simulink model "DQReferenceCurrentCalculationComponent"  (R2025b)
settings: Solver=FixedStepDiscrete  StartTime=0.0  StopTime=10.0  RelTol=1e-3
undefined symbols (not defined in the file): D1, P
settings Model: OrderFunctionsByDependency=on  Creator=dakaihu  LastModifiedBy=dakaihu
settings OptimizationCC: DefaultParameterBehavior=Inlined  UseFloatMulNetSlope=on  EnhancedBackFolding=on  PassReuseOutputArgsAs=Individual arguments  ZeroExternalMemoryAtStartup=off  ZeroInternalMemoryAtStartup=off  OptimizeBlockOrder=speed  DifferentSizesBufferReuse=on  OptimizationCustomize=off  EfficientTunableParamExpr=on
settings DebuggingCC: ParameterTunabilityLossMsg=error
settings HardwareCC: ProdBitPerChar=16.0  ProdBitPerInt=16.0  ProdBitPerPointer=32.0  ProdBitPerSizeT=32.0  ProdBitPerPtrDiffT=32.0  ProdLargestAtomicInteger=Integer  ProdLargestAtomicFloat=None  ProdWordSize=16.0  ProdLongLongMode=on  ProdHWDeviceType=Texas Instruments->C2000
settings SFSimCC: MATLABDynamicMemAlloc=off
settings RTWCC: SystemTargetFile=ert.tlc  GenCodeOnly=on  TemplateMakefile=ert_default_tmf  Description=Embedded Coder
settings CodeAppCC: ForceParamTrailComments=on  IgnoreCustomStorageClasses=off  MaxIdLength=60.0  OperatorAnnotations=on  SimulinkDataObjDesc=on  SFDataObjDesc=on  InsertBlockDesc=on
settings ERTTargetCC: ERTCustomFileTemplate=example_file_process.tlc  TargetLangStandard=C99 (ISO)  GenerateSampleERTMain=on

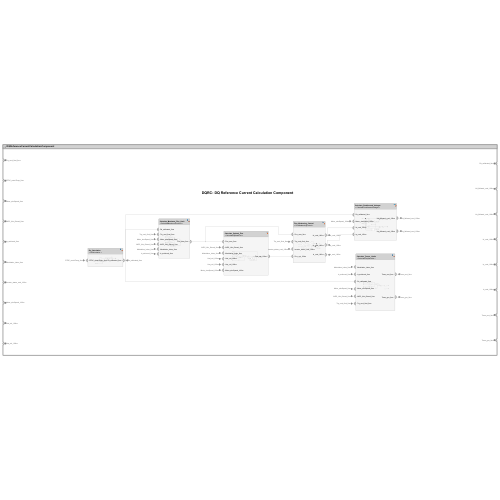
[thumbnail: Simulink's stored preview of the top-level diagram]
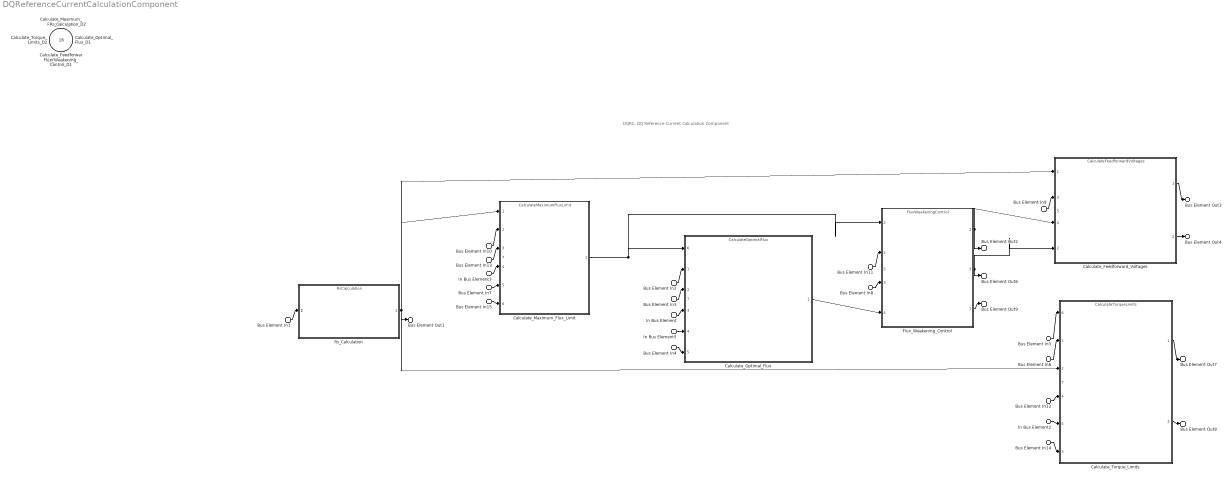
== system DQReferenceCurrentCalculationComponent ==
  note: DQRC: DQ Reference Current Calculation Component
  Bus Element In11 : Inport  RequirementInfo={} %GIDa_42953e8e_de57_4322_b6d3_fbe42e62adbf  PortName=Trq_cmd_final_2ms
  Bus Element In10 : Inport  RequirementInfo={} %GIDa_8c77aa49_9124_491b_8864_da37a441f5cb  PortName=Trq_cmd_final_2ms
  Bus Element In14 : Inport  RequirementInfo={} %GIDa_ea2f610a_4c5f_4cd4_9701_be585be16287  PortName=Trq_cmd_final_2ms
  Bus Element In1 : Inport  RequirementInfo={} %GIDa_4f0251a4_2495_47e1_b29c_9e0429a6851b  Port=2  PortName=STDC_motorTemp_2ms
  Bus Element In13 : Inport  RequirementInfo={} %GIDa_c753a603_7d00_42cf_be23_a4aecb64df4c  Port=3  PortName=Motor_elecSpeed_2ms
  Bus Element In12 : Inport  RequirementInfo={} %GIDa_cf1e9558_22e9_402c_a4b9_90f14ffe8b89  Port=3  PortName=Motor_elecSpeed_2ms
  In Bus Element3 : Inport  RequirementInfo={} %GIDa_41c1c28b_496d_4099_b24e_4d87927b0cd5  Port=4  PortName=IHDC_Vdc_filtered_2ms
  Bus Element In2 : Inport  RequirementInfo={} %GIDa_620fb42b_f1fb_400e_beea_66cdd1a5168a  Port=4  PortName=IHDC_Vdc_filtered_2ms
  In Bus Element2 : Inport  RequirementInfo={} %GIDa_a1449eb5_d98c_47be_a41f_d54f6146e101  Port=4  PortName=IHDC_Vdc_filtered_2ms
  Bus Element In6 : Inport  RequirementInfo={} %GIDa_46e95821_090d_4c5e_b6ae_42df5a77a427  Port=5  PortName=Is_achieved_2ms
  Bus Element In15 : Inport  RequirementInfo={} %GIDa_5aa52e8c_01f1_4417_9777_fe34b7f6ede0  Port=5  PortName=Is_achieved_2ms
  Bus Element In7 : Inport  RequirementInfo={} %GIDa_024a4306_83b0_46fe_af59_1f46b343fa8c  Port=6  PortName=Modulation_index_2ms
  Bus Element In3 : Inport  RequirementInfo={} %GIDa_be1195a5_2365_4ab0_90e8_c535b97f38fb  Port=6  PortName=Modulation_index_2ms
  Bus Element In5 : Inport  RequirementInfo={} %GIDa_dc760428_b6dc_4320_9a29_40c08d693f8a  Port=6  PortName=Modulation_index_2ms
  Bus Element In8 : Inport  RequirementInfo={} %GIDa_b12bee26_3679_4b52_8fa4_20643664e455  Port=7  PortName=Inverter_status_cmd_100us
  Bus Element In9 : Inport  RequirementInfo={} %GIDa_3f02f1c3_17f3_49f8_a464_eadd2057f829  Port=8  PortName=Motor_elecSpeed_100us
  Bus Element In4 : Inport  RequirementInfo={} %GIDa_8f5b8e9c_1d9d_4003_b734_3b70d64320b5  Port=8  PortName=Motor_elecSpeed_100us
  In Bus Element : Inport  RequirementInfo={} %GIDa_7ff0a437_48bf_41fa_8fef_4c1583c1267a  Port=9  PortName=Usd_ctrl_100us
  In Bus Element5 : Inport  RequirementInfo={} %GIDa_fb215a39_59d4_42c0_a18e_4b3e3a2c8f98  Port=10  PortName=Usq_ctrl_100us
  Calculate_Feedforward_Voltages_D1 : Inport  Port=11  OutputFunctionCall=on
  Calculate_Maximum_Flux_Limit_D2 : Inport  Port=12  OutputFunctionCall=on
  Calculate_Optimal_Flux_D1 : Inport  Port=13  OutputFunctionCall=on
  Calculate_Torque_Limits_D2 : Inport  Port=14  OutputFunctionCall=on
  Flux_Weakening_Control_D1 : Inport  Port=15  OutputFunctionCall=on
  Rs_Calculation_D2 : Inport  Port=16  OutputFunctionCall=on
  "Calculate_Feedforward_Voltages " : ModelReference  RequirementInfo={} %GIDa_c2d31358_4466_4952_b1b2_7ab47b6be7d3  ModelNameDialog=CalculateFeedforwardVoltages  SimulationMode=Normal  ScheduleRates=on  CachedPortDiscreteRates=[0.0001]  ModelEventPortInfo=P:D1[0.0001][0][0]  ModelReferenceVersion=2.2
      settings: PortSchema="{\"entries\":[{\"content\":{\"headerSize\":38,\"margin\":15,\"minimumSpacing\":25,\"sides\":[{\"content\":{\"connectorIds\":[\"In1\",\"In3\",\"In4\",\"In2\"]},\"type\":\"ConnectorPlacement.EquallySpacedRectSide\",\"uuid\":\"b2f30fca-3d8e-46ee-af1d-282b22b9b844\"},{\"content\":{\"connectorIds\":[\"Out1\",\"Out2\"],\"side\":\"RIGHT\"},\"type\":\"ConnectorPlacement.EquallySpacedRectSide\",\"uuid\":\"2d7d706d-eac4-4c73-84e8-2a36a393a616\"},{\"content\":{\"side\":\"TOP\"},\"type\":\"ConnectorPlacement.EquallySpacedRectSide\",\"uuid\":\"b52ae510-b7cc-4ed0-8d34-4a095deae41b\"},{\"content\":{\"side\":\"BOTTOM\"},\"type\":\"ConnectorPlacement.EquallySpacedRectSide\",\"uuid\":\"4f396a3e-469c-4bfe-8758-61b37cfc3b8b\"},{\"content\":{\"connectorIds\":[\"In5\"],\"side\":\"HIDDEN\"},\"type\":\"ConnectorPlacement.EquallySpacedRectSide\",\"uuid\":\"844b9219-0887-483b-96de-eb0af172b250\"}]},\"type\":\"ConnectorPlacement.EquallySpacedConnector\",\"uuid\":\"1257e7cc-1858-4bc4-ab05-7b00060cf0d5\"}],\"packageUris\":[\"http://schema.mathworks.com/mf0/Connector/R2020b\"],\"version\":\"1.0\"}"
  Calculate_Maximum_Flux_Limit : ModelReference  RequirementInfo={} %GIDa_a87a5d76_4785_45de_8980_7f650c5fa9a2  ModelNameDialog=CalculateMaximumFluxLimit  SimulationMode=Normal  ScheduleRates=on  CachedPortDiscreteRates=[0.002]  ModelEventPortInfo=P:D1[0.002][0][0]  ModelReferenceVersion=2.2
      settings: PortSchema="{\"entries\":[{\"content\":{\"headerSize\":38,\"margin\":15,\"minimumSpacing\":25,\"sides\":[{\"content\":{\"connectorIds\":[\"In1\",\"In2\",\"In3\",\"In4\",\"In5\",\"In6\"]},\"type\":\"ConnectorPlacement.EquallySpacedRectSide\",\"uuid\":\"b2f30fca-3d8e-46ee-af1d-282b22b9b844\"},{\"content\":{\"connectorIds\":[\"Out1\"],\"side\":\"RIGHT\"},\"type\":\"ConnectorPlacement.EquallySpacedRectSide\",\"uuid\":\"2d7d706d-eac4-4c73-84e8-2a36a393a616\"},{\"content\":{\"side\":\"TOP\"},\"type\":\"ConnectorPlacement.EquallySpacedRectSide\",\"uuid\":\"b52ae510-b7cc-4ed0-8d34-4a095deae41b\"},{\"content\":{\"connectorIds\":[\"In7\"],\"side\":\"HIDDEN\"},\"type\":\"ConnectorPlacement.EquallySpacedRectSide\",\"uuid\":\"d71c0094-66e8-4c46-a453-bb528cb08d1e\"}]},\"type\":\"ConnectorPlacement.EquallySpacedConnector\",\"uuid\":\"1257e7cc-1858-4bc4-ab05-7b00060cf0d5\"}],\"packageUris\":[\"http://schema.mathworks.com/mf0/Connector/R2020b\"],\"version\":\"1.0\"}"
  Calculate_Optimal_Flux : ModelReference  RequirementInfo={} %GIDa_8fb845d2_dc36_4fd4_9091_e75f493b384f  ModelNameDialog=CalculateOptimalFlux  SimulationMode=Normal  ScheduleRates=on  CachedPortDiscreteRates=[0.0001]  ModelEventPortInfo=P:D1[0.0001][0][0]  ModelReferenceVersion=2.2
      settings: PortSchema="{\"entries\":[{\"content\":{\"headerSize\":38,\"margin\":15,\"minimumSpacing\":25,\"sides\":[{\"content\":{\"connectorIds\":[\"In6\",\"In1\",\"In2\",\"In3\",\"In4\",\"In5\"]},\"type\":\"ConnectorPlacement.EquallySpacedRectSide\",\"uuid\":\"b2f30fca-3d8e-46ee-af1d-282b22b9b844\"},{\"content\":{\"connectorIds\":[\"Out1\"],\"side\":\"RIGHT\"},\"type\":\"ConnectorPlacement.EquallySpacedRectSide\",\"uuid\":\"2d7d706d-eac4-4c73-84e8-2a36a393a616\"},{\"content\":{\"side\":\"TOP\"},\"type\":\"ConnectorPlacement.EquallySpacedRectSide\",\"uuid\":\"b52ae510-b7cc-4ed0-8d34-4a095deae41b\"},{\"content\":{\"connectorIds\":[\"In7\"],\"side\":\"HIDDEN\"},\"type\":\"ConnectorPlacement.EquallySpacedRectSide\",\"uuid\":\"a73ad583-9615-4874-ab2d-c98618391765\"}]},\"type\":\"ConnectorPlacement.EquallySpacedConnector\",\"uuid\":\"1257e7cc-1858-4bc4-ab05-7b00060cf0d5\"}],\"packageUris\":[\"http://schema.mathworks.com/mf0/Connector/R2020b\"],\"version\":\"1.0\"}"
  Calculate_Torque_Limits : ModelReference  RequirementInfo={} %GIDa_739b0719_e4db_4236_85d1_8411d06b7a29  ModelNameDialog=CalculateTorqueLimits  SimulationMode=Normal  ScheduleRates=on  CachedPortDiscreteRates=[0.002]  ModelEventPortInfo=P:D1[0.002][0][0]  ModelReferenceVersion=2.2
      settings: PortSchema="{\"entries\":[{\"content\":{\"headerSize\":38,\"margin\":15,\"minimumSpacing\":25,\"sides\":[{\"content\":{\"connectorIds\":[\"In6\",\"In1\",\"In2\",\"In4\",\"In5\",\"In3\"]},\"type\":\"ConnectorPlacement.EquallySpacedRectSide\",\"uuid\":\"b2f30fca-3d8e-46ee-af1d-282b22b9b844\"},{\"content\":{\"connectorIds\":[\"Out1\",\"Out2\"],\"side\":\"RIGHT\"},\"type\":\"ConnectorPlacement.EquallySpacedRectSide\",\"uuid\":\"2d7d706d-eac4-4c73-84e8-2a36a393a616\"},{\"content\":{\"side\":\"TOP\"},\"type\":\"ConnectorPlacement.EquallySpacedRectSide\",\"uuid\":\"b52ae510-b7cc-4ed0-8d34-4a095deae41b\"},{\"content\":{\"connectorIds\":[\"In7\"],\"side\":\"HIDDEN\"},\"type\":\"ConnectorPlacement.EquallySpacedRectSide\",\"uuid\":\"bfe6c03f-982a-4b44-9f69-90b5c2e623cb\"}]},\"type\":\"ConnectorPlacement.EquallySpacedConnector\",\"uuid\":\"1257e7cc-1858-4bc4-ab05-7b00060cf0d5\"}],\"packageUris\":[\"http://schema.mathworks.com/mf0/Connector/R2020b\"],\"version\":\"1.0\"}"
  Flux_Weakening_Control : ModelReference  RequirementInfo={} %GIDa_9fe039aa_e028_435b_8ff1_3eb9542dc048  ModelNameDialog=FluxWeakeningControl  SimulationMode=Normal  ScheduleRates=on  CachedPortDiscreteRates=[0.0001]  ModelEventPortInfo=P:D1[0.0001][0][0]  ModelReferenceVersion=2.0
      settings: PortSchema="{\"entries\":[{\"content\":{\"headerSize\":38,\"margin\":15,\"minimumSpacing\":25,\"sides\":[{\"content\":{\"connectorIds\":[\"In2\",\"In1\",\"In3\",\"In4\"]},\"type\":\"ConnectorPlacement.EquallySpacedRectSide\",\"uuid\":\"b2f30fca-3d8e-46ee-af1d-282b22b9b844\"},{\"content\":{\"connectorIds\":[\"Out2\",\"Out3\",\"Out1\"],\"side\":\"RIGHT\"},\"type\":\"ConnectorPlacement.EquallySpacedRectSide\",\"uuid\":\"2d7d706d-eac4-4c73-84e8-2a36a393a616\"},{\"content\":{\"side\":\"TOP\"},\"type\":\"ConnectorPlacement.EquallySpacedRectSide\",\"uuid\":\"b52ae510-b7cc-4ed0-8d34-4a095deae41b\"},{\"content\":{\"connectorIds\":[\"In5\"],\"side\":\"HIDDEN\"},\"type\":\"ConnectorPlacement.EquallySpacedRectSide\",\"uuid\":\"7d4a66f0-dbef-49ea-acd8-9a102931ed07\"}]},\"type\":\"ConnectorPlacement.EquallySpacedConnector\",\"uuid\":\"1257e7cc-1858-4bc4-ab05-7b00060cf0d5\"}],\"packageUris\":[\"http://schema.mathworks.com/mf0/Connector/R2020b\"],\"version\":\"1.0\"}"
  Rs_Calculation : ModelReference  RequirementInfo={} %GIDa_2e11c86d_9488_40ba_9db8_781f3426afdc  ModelNameDialog=RsCalculation  SimulationMode=Normal  ScheduleRates=on  CachedPortDiscreteRates=[0.002]  ModelEventPortInfo=P:D1[0.002][0][0]  ModelReferenceVersion=3.0
      settings: PortSchema="{\"entries\":[{\"content\":{\"headerSize\":38,\"margin\":15,\"minimumSpacing\":25,\"sides\":[{\"content\":{\"connectorIds\":[\"In1\"]},\"type\":\"ConnectorPlacement.EquallySpacedRectSide\",\"uuid\":\"b2f30fca-3d8e-46ee-af1d-282b22b9b844\"},{\"content\":{\"connectorIds\":[\"Out1\"],\"side\":\"RIGHT\"},\"type\":\"ConnectorPlacement.EquallySpacedRectSide\",\"uuid\":\"2d7d706d-eac4-4c73-84e8-2a36a393a616\"},{\"content\":{\"side\":\"TOP\"},\"type\":\"ConnectorPlacement.EquallySpacedRectSide\",\"uuid\":\"b52ae510-b7cc-4ed0-8d34-4a095deae41b\"},{\"content\":{\"connectorIds\":[\"In2\"],\"side\":\"HIDDEN\"},\"type\":\"ConnectorPlacement.EquallySpacedRectSide\",\"uuid\":\"e9258453-274e-42d5-b20b-278cbee769f2\"}]},\"type\":\"ConnectorPlacement.EquallySpacedConnector\",\"uuid\":\"1257e7cc-1858-4bc4-ab05-7b00060cf0d5\"}],\"packageUris\":[\"http://schema.mathworks.com/mf0/Connector/R2020b\"],\"version\":\"1.0\"}"
  Bus Element Out1 : Outport  RequirementInfo={} %GIDa_5c6ca521_ec0b_44c3_8d07_578d6b9f1c60  PortName=Rs_calibrated_2ms
  Bus Element Out3 : Outport  RequirementInfo={} %GIDa_7d6f6061_9fcc_414c_968c_ee7b380f3c52  Port=2  PortName=Ud_fdfrward_cmd_100us
  Bus Element Out4 : Outport  RequirementInfo={} %GIDa_694c25c9_4840_4d45_8c78_c66e7d74dff2  Port=3  PortName=Uq_fdfrward_cmd_100us
  Bus Element Out2 : Outport  RequirementInfo={} %GIDa_de25d3e3_44c5_485b_a095_a8d9b9fb7d3b  Port=4  PortName=Id_cmd_100us
  Bus Element Out6 : Outport  RequirementInfo={} %GIDa_c159c7b9_5d90_4cf6_bfd9_5456d3df1725  Port=5  PortName=Iq_cmd_100us
  Bus Element Out9 : Outport  RequirementInfo={} %GIDa_7ebf1886_4633_46e5_8be8_afa35ed6b1ba  Port=6  PortName=Is_cmd_100us
  Bus Element Out7 : Outport  RequirementInfo={} %GIDa_0926f624_5632_4be0_b2a9_1bf1a45cf719  Port=7  PortName=Tmax_mot_2ms
  Bus Element Out8 : Outport  RequirementInfo={} %GIDa_70777ce8_9636_4637_aa0f_a3c244b1ff29  Port=8  PortName=Tmax_gen_2ms
  wires:
  "Calculate_Feedforward_Voltages "/1 -> Bus Element Out3/1
  Bus Element In10/1 -> Calculate_Maximum_Flux_Limit/2
  Bus Element In11/1 -> Flux_Weakening_Control/1
  Calculate_Torque_Limits/1 -> Bus Element Out7/1
  Calculate_Torque_Limits/2 -> Bus Element Out8/1
  Bus Element In3/1 -> Calculate_Optimal_Flux/2
  Calculate_Optimal_Flux/1 -> Flux_Weakening_Control/4
  Bus Element In15/1 -> Calculate_Maximum_Flux_Limit/6
  Bus Element In13/1 -> Calculate_Maximum_Flux_Limit/3
  In Bus Element5/1 -> Calculate_Optimal_Flux/4
  Bus Element In12/1 -> Calculate_Torque_Limits/4
  In Bus Element/1 -> Calculate_Optimal_Flux/3
  In Bus Element2/1 -> Calculate_Torque_Limits/5
  Bus Element In2/1 -> Calculate_Optimal_Flux/1
  "Calculate_Feedforward_Voltages "/2 -> Bus Element Out4/1
  Bus Element In9/1 -> "Calculate_Feedforward_Voltages "/3
  Flux_Weakening_Control/1 -> Bus Element Out9/1
  In Bus Element3/1 -> Calculate_Maximum_Flux_Limit/4
  Bus Element In4/1 -> Calculate_Optimal_Flux/5
  Bus Element In5/1 -> Calculate_Torque_Limits/6
  Bus Element In14/1 -> Calculate_Torque_Limits/3
  Bus Element In8/1 -> Flux_Weakening_Control/3
  Bus Element In1/1 -> Rs_Calculation/1
  Flux_Weakening_Control/3 -> Bus Element Out6/1, "Calculate_Feedforward_Voltages "/2
  Bus Element In6/1 -> Calculate_Torque_Limits/1
  Flux_Weakening_Control/2 -> Bus Element Out2/1, "Calculate_Feedforward_Voltages "/4
  Rs_Calculation/1 -> Calculate_Torque_Limits/2, Bus Element Out1/1, Calculate_Maximum_Flux_Limit/1, "Calculate_Feedforward_Voltages "/1
  Bus Element In7/1 -> Calculate_Maximum_Flux_Limit/5
  Calculate_Maximum_Flux_Limit/1 -> Calculate_Optimal_Flux/6, Flux_Weakening_Control/2
